simulink model "lab8"  (R2023b)
settings: Solver=VariableStepAuto  StartTime=0.0  StopTime=1000  RelTol=1e-3
values from neighbouring files (symbols this model uses):
  init_ss = 1    [init.m]
  k_0 = 1    [init.m]
  k_M_0 = 6    [init.m]
  k_M_1 = 5    [init.m]
undefined symbols (not defined in the file or in its folder): Ass, Bss, Css, Dss
settings Model: Creator=vladislav  LastModifiedBy=lalayants
settings RTWCC: GPUComputeCapability=5.0

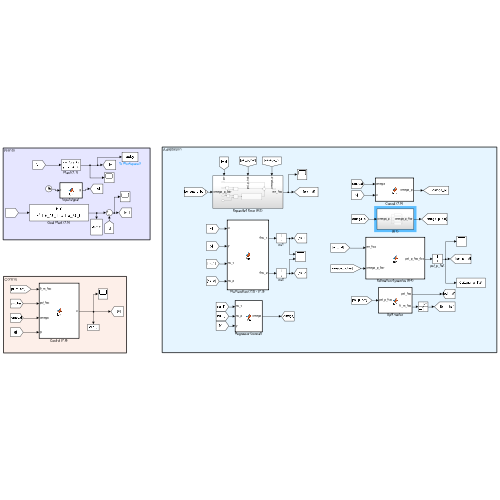
[thumbnail: Simulink's stored preview of the top-level diagram]
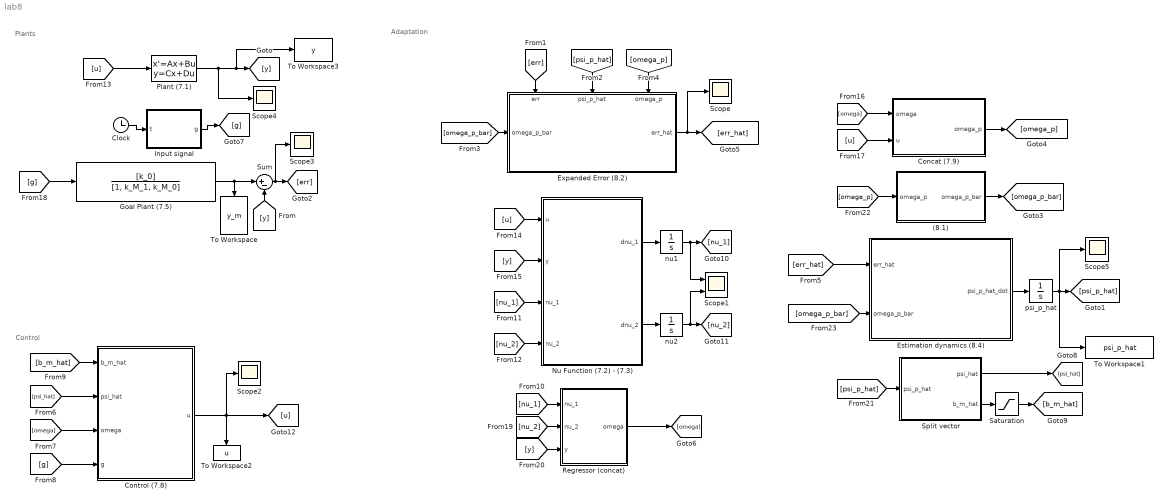
== system lab8 ==
  note: Control
  note: Adaptation
  note: Plants
  (8.1) : Subsystem
  Clock : Clock
  Concat (7.9) : MATLAB Function  TreatAsAtomicUnit=on
  Control (7.8) : MATLAB Function  TreatAsAtomicUnit=on
  Estimation dynamics (8.4) : MATLAB Function  TreatAsAtomicUnit=on
  Expanded Error (8.2) : Subsystem
      settings: PortSchema="{\"entries\":[{\"content\":{\"sides\":[{\"content\":{\"connectorIds\":[\"In1\"]},\"type\":\"ConnectorPlacement.EquallySpacedRectSide\",\"uuid\":\"8352c707-0f0f-4965-ab9a-a54854278a50\"},{\"content\":{\"connectorIds\":[\"Out1\"],\"side\":\"RIGHT\"},\"type\":\"ConnectorPlacement.EquallySpacedRectSide\",\"uuid\":\"2870c956-d2c8-4da6-8e00-d09a3c8192c5\"},{\"content\":{\"connectorIds\":[\"In2\",\"In3\",\"In4\"],\"side\":\"TOP\"},\"type\":\"ConnectorPlacement.EquallySpacedRectSide\",\"uuid\":\"24a49dbe-8490-4683-b6bd-eeeb5ddd82cb\"}]},\"type\":\"ConnectorPlacement.EquallySpacedConnector\",\"uuid\":\"a465fb68-7205-42f4-9068-d6b504ebde08\"}],\"packageUris\":[\"http://schema.mathworks.com/mf0/Connector/R2020b\"],\"version\":\"1.0\"}"
  Goal Plant (7.5) : TransferFcn  Numerator=[k_0]  Denominator=[1, k_M_1, k_M_0]
  Input signal : MATLAB Function  TreatAsAtomicUnit=on
  Nu Function (7.2) - (7.3) : MATLAB Function  TreatAsAtomicUnit=on
  Plant (7.1) : StateSpace  A=Ass  B=Bss  C=Css  D=Dss  InitialCondition=init_ss
  Regressor (concat) : MATLAB Function  TreatAsAtomicUnit=on
  Saturation : Saturate  UpperLimit=10000000  LowerLimit=0.1
  Scope{,2..5} (5 alike) : Scope
  Scope1 : Scope  NumInputPorts=2
  Split vector : MATLAB Function  TreatAsAtomicUnit=on
  Sum : Sum  Inputs=|+-
  To Workspace : ToWorkspace  VariableName=y_m  SaveFormat=Timeseries  SampleTime=-1
  To Workspace1 : ToWorkspace  VariableName=psi_p_hat  SaveFormat=Timeseries  SampleTime=-1
  To Workspace2 : ToWorkspace  VariableName=u  SaveFormat=Timeseries  SampleTime=-1
  To Workspace3 : ToWorkspace  VariableName=y  SaveFormat=Timeseries  SampleTime=-1
  nu1 : Integrator
  nu2 : Integrator
  psi_p_hat : Integrator  InitialCondition=[10;10;10;10]
  wires:
  Nu Function (7.2) - (7.3)/1(dnu_1) -> nu1/1
  Nu Function (7.2) - (7.3)/2(dnu_2) -> nu2/1
  nu2/1 -> Scope1/2, [nu_2]
  nu1/1 -> Scope1/1, [nu_1]
  Control (7.8)/1(u) -> Scope2/1, [u], To Workspace2/1
  Regressor (concat)/1(omega) -> [omega]
  Concat (7.9)/1(omega_p) -> [omega_p]
  Estimation dynamics (8.4)/1(psi_p_hat_dot) -> psi_p_hat/1
  (8.1)/1(omega_p_bar) -> [omega_p_bar]
  Goal Plant (7.5)/1 -> To Workspace/1, Sum/1
  [y] -> Sum/2
  Sum/1 -> Scope3/1, [err]
  [err] -> Expanded Error (8.2)/2(err)
  psi_p_hat/1 -> To Workspace1/1, Scope5/1, [psi_p_hat]
  [psi_p_hat] -> Expanded Error (8.2)/3(psi_p_hat)
  [omega_p_bar] -> Expanded Error (8.2)/1(omega_p_bar)
  [omega_p] -> Expanded Error (8.2)/4(omega_p)
  Expanded Error (8.2)/1(err_hat) -> Scope/1, [err_hat]
  [err_hat] -> Estimation dynamics (8.4)/1(err_hat)
  [omega] -> Control (7.8)/3(omega)
  [g] -> Control (7.8)/4(g)
  Split vector/1(psi_hat) -> [psi_hat]
  [psi_hat] -> Control (7.8)/2(psi_hat)
  [b_m_hat] -> Control (7.8)/1(b_m_hat)
  Split vector/2(b_m_hat) -> Saturation/1
  Saturation/1 -> [b_m_hat]
  [nu_1] -> Nu Function (7.2) - (7.3)/3(nu_1)
  [nu_2] -> Nu Function (7.2) - (7.3)/4(nu_2)
  [u] -> Nu Function (7.2) - (7.3)/1(u)
  [y] -> Nu Function (7.2) - (7.3)/2(y)
  [omega] -> Concat (7.9)/1(omega)
  [u] -> Concat (7.9)/2(u)
  [g] -> Goal Plant (7.5)/1
  Input signal/1(g) -> [g]
  Clock/1 -> Input signal/1(t)
  [nu_1] -> Regressor (concat)/1(nu_1)
  [nu_2] -> Regressor (concat)/2(nu_2)
  [y] -> Regressor (concat)/3(y)
  [psi_p_hat] -> Split vector/1(psi_p_hat)
  [omega_p] -> (8.1)/1(omega_p)
  [omega_p_bar] -> Estimation dynamics (8.4)/2(omega_p_bar)
  [u] -> Plant (7.1)/1
  Plant (7.1)/1 -> Scope4/1, To Workspace3/1, [y]

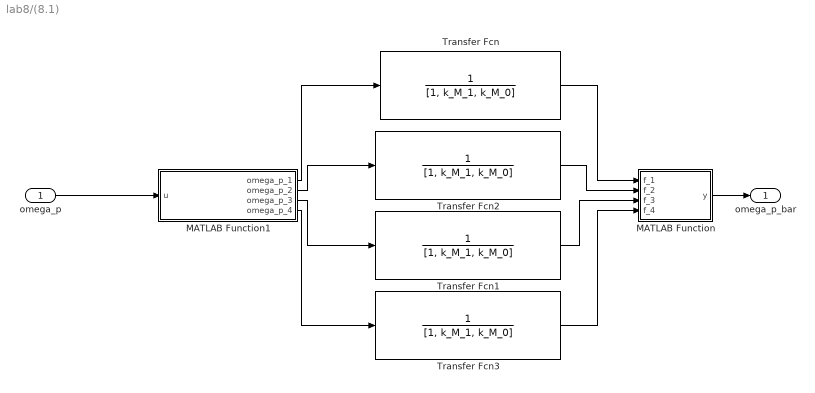
== system lab8/(8.1) ==
  omega_p : Inport
  MATLAB Function : MATLAB Function  TreatAsAtomicUnit=on
  MATLAB Function1 : MATLAB Function  TreatAsAtomicUnit=on
  Transfer Fcn{,1..3} (4 alike) : TransferFcn  Denominator=[1, k_M_1, k_M_0]
  omega_p_bar : Outport
  wires:
  Transfer Fcn2/1 -> MATLAB Function/2(f_2)
  Transfer Fcn1/1 -> MATLAB Function/3(f_3)
  Transfer Fcn/1 -> MATLAB Function/1(f_1)
  MATLAB Function/1(y) -> omega_p_bar/1
  omega_p/1 -> MATLAB Function1/1(u)
  MATLAB Function1/2(omega_p_2) -> Transfer Fcn2/1
  MATLAB Function1/1(omega_p_1) -> Transfer Fcn/1
  MATLAB Function1/3(omega_p_3) -> Transfer Fcn1/1
  MATLAB Function1/4(omega_p_4) -> Transfer Fcn3/1
  Transfer Fcn3/1 -> MATLAB Function/4(f_4)

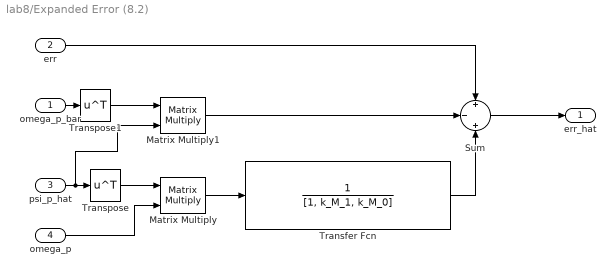
== system lab8/Expanded Error (8.2) ==
  omega_p_bar : Inport
  err : Inport  Port=2
  psi_p_hat : Inport  Port=3
  omega_p : Inport  Port=4
  Matrix Multiply : Product  Multiplication=Matrix(*)
  Matrix Multiply1 : Product  Multiplication=Matrix(*)
  Sum : Sum  Inputs=+|-|+
  Transfer Fcn : TransferFcn  Denominator=[1, k_M_1, k_M_0]
  Transpose : Math  Operator=transpose
  Transpose1 : Math  Operator=transpose
  err_hat : Outport
  wires:
  Transpose/1 -> Matrix Multiply/1
  omega_p/1 -> Matrix Multiply/2
  Matrix Multiply/1 -> Transfer Fcn/1
  omega_p_bar/1 -> Transpose1/1
  Transpose1/1 -> Matrix Multiply1/1
  psi_p_hat/1 -> Matrix Multiply1/2, Transpose/1
  Transfer Fcn/1 -> Sum/3
  Matrix Multiply1/1 -> Sum/2
  err/1 -> Sum/1
  Sum/1 -> err_hat/1

== matlab function lab8/Control (7.8) ==
  data: b_m_hat input; u output; psi_hat input; omega input; g input; k_0 parameter
function u = fcn(b_m_hat, psi_hat, omega, g, k_0)

u = (-psi_hat' * omega + k_0 * g) / b_m_hat;

== matlab function lab8/Nu Function (7.2) - (7.3) ==
  data: u input; dnu_1 output; y input; nu_1 input; nu_2 input; dnu_2 output; Lambda parameter
function [dnu_1, dnu_2] = fcn(u, y, nu_1, nu_2, Lambda)

dnu_1 = Lambda*nu_1 + u;
dnu_2 = Lambda*nu_2 + y;

== matlab function lab8/Regressor (concat) ==
  data: nu_1 input; omega output; nu_2 input; y input
function omega = fcn(nu_1, nu_2, y)

omega = [nu_1; nu_2; y];

== matlab function lab8/(8.1)/MATLAB Function ==
  data: f_1 input; y output; f_2 input; f_3 input; f_4 input
function y = fcn(f_1, f_2, f_3, f_4)

y = [f_1; f_2; f_3; f_4];

== matlab function lab8/(8.1)/MATLAB Function1 ==
  data: u input; omega_p_1 output; omega_p_2 output; omega_p_3 output; omega_p_4 output
function [omega_p_1, omega_p_2, omega_p_3, omega_p_4] = fcn(u)

omega_p_1 = u(1);
omega_p_2 = u(2);
omega_p_3 = u(3);
omega_p_4 = u(4);

== matlab function lab8/Concat (7.9) ==
  data: omega input; u input; omega_p output
function omega_p = fcn(omega, u)

omega_p = [-omega(1); -omega(2); -omega(3); -u];

== matlab function lab8/Estimation dynamics (8.4) ==
  data: err_hat input; psi_p_hat_dot output; omega_p_bar input; gamma parameter
function psi_p_hat_dot = fcn(err_hat, omega_p_bar, gamma)

psi_p_hat_dot = gamma*omega_p_bar * err_hat / (1 + omega_p_bar' * omega_p_bar); % Assuming Г = id

== matlab function lab8/Input signal ==
  data: t input; g output
function g = fcn(t)

g = 7 * cos(3 * t + 2) + 8 ;

== matlab function lab8/Split vector ==
  data: psi_p_hat input; psi_hat output; b_m_hat output
function [psi_hat, b_m_hat] = fcn(psi_p_hat)

b_m_hat = psi_p_hat(4,1);
psi_hat = psi_p_hat(1:3,1);
